simulink model "signal_analysis"  (R2019a)
settings: Solver=FixedStepDiscrete  StartTime=0.0  StopTime=inf  RelTol=1e-3
StartFcn:
  | default_path = fileread('.\temp\dataPath.txt');
  | [file, path] = uigetfile([default_path,'\*.dat'], '选择GPS数据文件');
  | if file==0
  |     error('Invalid file!')
  | end
  | if strcmp(file(1:4),'B210')==0 && strcmp(file(1:5),'PLUTO')==0
  |     error('File error!')
  | end
  | file_path = [path, file];
StopFcn:
  | clearvars default_path file path file_path
libraries: dspsrcs4 x1
settings Model: Creator=longt  LastModifiedBy=longt
settings DataIOCC: SaveOutput=off  SignalLogging=off  DSMLogging=off  SaveTime=off  ReturnWorkspaceOutputs=off

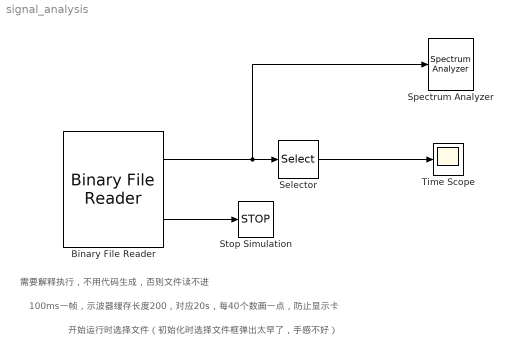
== system signal_analysis ==
  note: 开始运行时选择文件（初始化时选择文件框弹出太早了，手感不好）
  note: 100ms一帧，示波器缓存长度200，对应20s，每40个数画一点，防止显示卡
  note: 需要解释执行，不用代码生成，否则文件读不进
  Binary File Reader : dspsrcs4/Binary File Reader  Filename=file_path  HeaderStructure=struct([])  DataType=int16  SamplesPerFrame=4e5  IsDataComplex=on  NumChannels=1  OutputEOF=on  SampleTime=1/4e6  SimulateUsing=Interpreted execution
      settings: SourceProductName=DSP System Toolbox  SourceProductBaseCode=DS
  Selector : Selector  NumberOfDimensions=2  InputPortWidth=3  IndexOptions=Index vector (dialog),Index vector (dialog)  Indices=(1:10000)*40,1  OutputSizes=1,1
  Spectrum Analyzer : SpectrumAnalyzer
  Stop Simulation : Stop
  Time Scope : Scope
  wires:
  Binary File Reader/2 -> Stop Simulation/1
  Binary File Reader/1 -> Spectrum Analyzer/1, Selector/1
  Selector/1 -> Time Scope/1
